simulink model "DS3or"  (R2023a)
settings: Solver=VariableStepAuto  StartTime=0.0  StopTime=tsim  RelTol=1e-3
undefined symbols (not defined in the file): comp_noise_rms, comp_offset, fclk, fin, fs, OSR, pf1, pf2, pf3, ps1, ps2, ps3, q1, q2, q3, VDD, Vin_amp, Vin_cm, Vin_DC, Vref, VSS, W
settings Model: Creator=amantilla  LastModifiedBy=alexm
settings SolverCC: AlgebraicLoopSolver=TrustRegion
settings DebuggingCC: UnconnectedInputMsg=warning  UnconnectedOutputMsg=warning  UnconnectedLineMsg=warning
settings ModelReferenceCC: EnableRefExpFcnMdlSchedulingChecks=on
settings RTWCC: DLArmComputeVersion=19.05

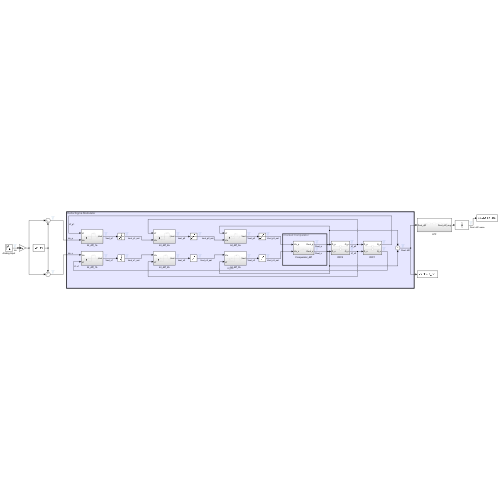
[thumbnail: Simulink's stored preview of the top-level diagram]
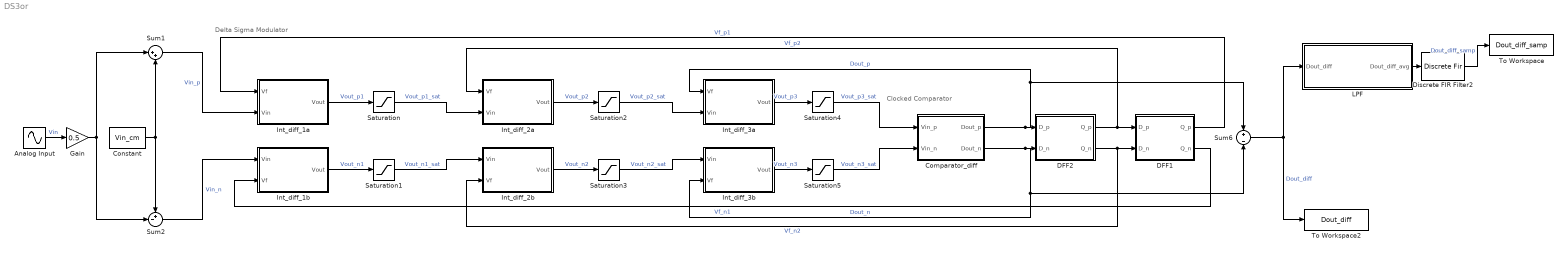
== system DS3or ==
  note: Delta Sigma Modulator
  note: Clocked Comparator
  Analog Input : Sin  Amplitude=Vin_amp  Bias=Vin_DC  Frequency=2*pi*fin  SampleTime=1/(fclk)
  Comparator_diff : Subsystem
  Constant : Constant  Value=Vin_cm
  DFF1 : Subsystem
  DFF2 : Subsystem
  Discrete FIR Filter2 : DiscreteFir  Coefficients=1  InitialStates=(VDD - VSS)/2  SampleTime=1/(fs)
  Gain : Gain  Gain=0.5
  Int_diff_1a : Subsystem
  Int_diff_1b : Subsystem
  Int_diff_2a : Subsystem
  Int_diff_2b : Subsystem
  Int_diff_3a : Subsystem
  Int_diff_3b : Subsystem
  LPF : Subsystem
  Saturation{,1..5} (6 alike) : Saturate  UpperLimit=0.9  LowerLimit=0
  Sum1 : Sum  Inputs=|++
  Sum2 : Sum  Inputs=+-|
  Sum6 : Sum  Inputs=+|-
  To Workspace : ToWorkspace  VariableName=Dout_diff_samp  SaveFormat=Timeseries  SampleTime=1/fs
  To Workspace2 : ToWorkspace  VariableName=Dout_diff  SaveFormat=Timeseries  SampleTime=1/fclk
  wires:
  Constant/1 -> Sum1/2, Sum2/1
  Sum6/1 -> To Workspace2/1, LPF/1(Dout_diff)  "Dout_diff"
  Gain/1 -> Sum2/2, Sum1/1
  Discrete FIR Filter2/1 -> To Workspace/1  "Dout_diff_samp"
  Sum2/1 -> Int_diff_1b/1(Vin)  "Vin_n"
  Int_diff_2b/1(Vout) -> Saturation3/1  "Vout_n2"
  Analog Input/1 -> Gain/1  "Vin"
  Sum1/1 -> Int_diff_1a/2(Vin)  "Vin_p"
  Int_diff_2a/1(Vout) -> Saturation2/1  "Vout_p2"
  Int_diff_1a/1(Vout) -> Saturation/1  "Vout_p1"
  Int_diff_1b/1(Vout) -> Saturation1/1  "Vout_n1"
  DFF1/1(Q_p) -> Int_diff_1a/1(Vf)  "Vf_p1"
  DFF1/2(Q_n) -> Int_diff_1b/2(Vf)  "Vf_n1"
  Comparator_diff/1(Dout_p) -> Sum6/1, Int_diff_3a/1(Vf), DFF2/1(D_p)  "Dout_p"
  Comparator_diff/2(Dout_n) -> Sum6/2, Int_diff_3b/2(Vf), DFF2/2(D_n)  "Dout_n"
  Saturation/1 -> Int_diff_2a/2(Vin)  "Vout_p1_sat"
  Saturation1/1 -> Int_diff_2b/1(Vin)  "Vout_n1_sat"
  Saturation2/1 -> Int_diff_3a/2(Vin)  "Vout_p2_sat"
  Saturation3/1 -> Int_diff_3b/1(Vin)  "Vout_n2_sat"
  DFF2/1(Q_p) -> DFF1/1(D_p), Int_diff_2a/1(Vf)  "Vf_p2"
  DFF2/2(Q_n) -> DFF1/2(D_n), Int_diff_2b/2(Vf)  "Vf_n2"
  Int_diff_3b/1(Vout) -> Saturation5/1  "Vout_n3"
  Int_diff_3a/1(Vout) -> Saturation4/1  "Vout_p3"
  Saturation4/1 -> Comparator_diff/1(Vin_p)  "Vout_p3_sat"
  Saturation5/1 -> Comparator_diff/2(Vin_n)  "Vout_n3_sat"
  LPF/1(Dout_diff_avg) -> Discrete FIR Filter2/1

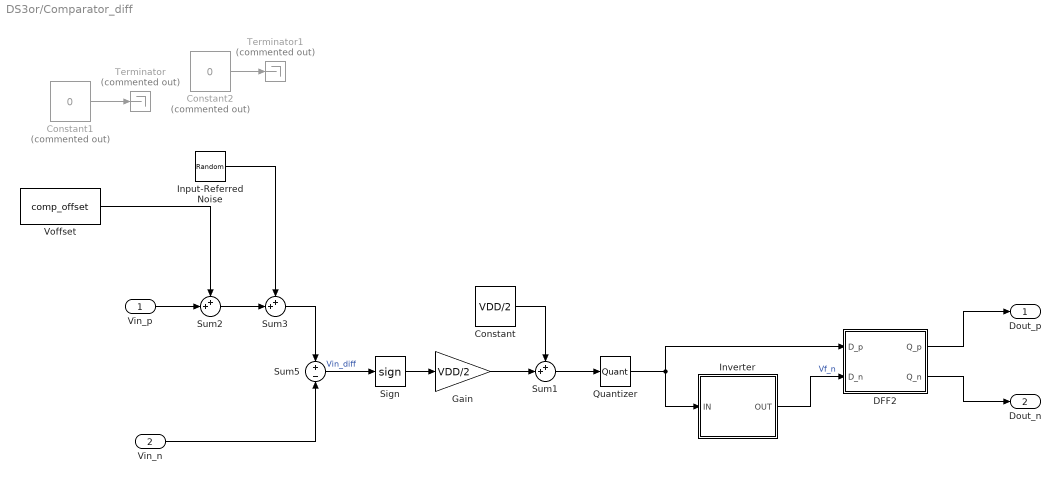
== system DS3or/Comparator_diff ==
  Vin_p : Inport
  Vin_n : Inport  Port=2
  Constant : Constant  Value=VDD/2  VectorParams1D=off  SampleTime=-1
  Constant1 : Constant  Commented=on  Value=0  VectorParams1D=off  SampleTime=-1
  Constant2 : Constant  Commented=on  Value=0  VectorParams1D=off  SampleTime=-1
  DFF2 : Subsystem
  Gain : Gain  Gain=VDD/2
  Input-Referred Noise : RandomNumber  Variance=comp_noise_rms  SampleTime=1/(4*fclk)
  Inverter : Subsystem
  Quantizer : Quantizer  QuantizationInterval=(VDD-VSS)
  Sign : Signum
  Sum1 : Sum  Inputs=++|
  Sum2 : Sum  Inputs=++|
  Sum3 : Sum  Inputs=++|
  Sum5 : Sum  Inputs=+|-
  Terminator : Terminator  Commented=on
  Terminator1 : Terminator  Commented=on
  Voffset : Constant  Value=comp_offset  VectorParams1D=off  SampleTime=-1
  Dout_p : Outport
  Dout_n : Outport  Port=2
  wires:
  Sum5/1 -> Sign/1  "Vin_diff"
  Vin_n/1 -> Sum5/2
  Sign/1 -> Gain/1
  Gain/1 -> Sum1/2
  Sum1/1 -> Quantizer/1
  Constant/1 -> Sum1/1
  Inverter/1(OUT) -> DFF2/2(D_n)  "Vf_n"
  Quantizer/1 -> Inverter/1(IN), DFF2/1(D_p)
  DFF2/1(Q_p) -> Dout_p/1
  DFF2/2(Q_n) -> Dout_n/1
  Vin_p/1 -> Sum2/2
  Sum2/1 -> Sum3/2
  Sum3/1 -> Sum5/1
  Constant1/1 -> Terminator/1
  Constant2/1 -> Terminator1/1
  Input-Referred Noise/1 -> Sum3/1
  Voffset/1 -> Sum2/1

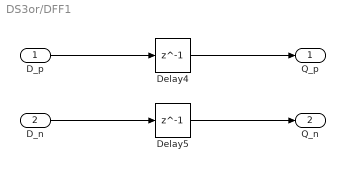
== system DS3or/DFF1 ==
  D_p : Inport
  D_n : Inport  Port=2
  Delay4 : Delay  DelayLength=1  InitialCondition=VSS  SampleTime=1/(fclk)
  Delay5 : Delay  DelayLength=1  InitialCondition=VDD  SampleTime=1/(fclk)
  Q_p : Outport
  Q_n : Outport  Port=2
  wires:
  Delay4/1 -> Q_p/1
  D_p/1 -> Delay4/1
  Delay5/1 -> Q_n/1
  D_n/1 -> Delay5/1

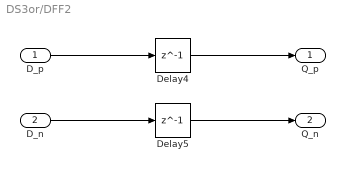
== system DS3or/DFF2 ==
  D_p : Inport
  D_n : Inport  Port=2
  Delay4 : Delay  DelayLength=1  InitialCondition=VSS  SampleTime=1/(fclk)
  Delay5 : Delay  DelayLength=1  InitialCondition=VDD  SampleTime=1/(fclk)
  Q_p : Outport
  Q_n : Outport  Port=2
  wires:
  Delay4/1 -> Q_p/1
  D_p/1 -> Delay4/1
  Delay5/1 -> Q_n/1
  D_n/1 -> Delay5/1

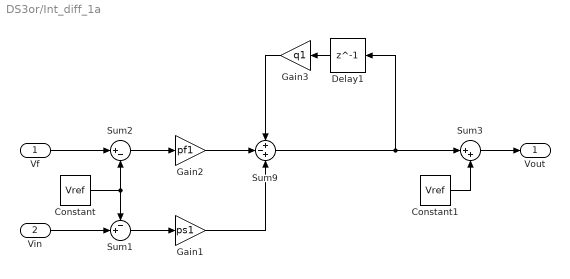
== system DS3or/Int_diff_1a ==
  Vf : Inport
  Vin : Inport  Port=2
  Constant : Constant  Value=Vref
  Constant1 : Constant  Value=Vref
  Delay1 : Delay  DelayLength=1  SampleTime=1/(fclk)
  Gain1 : Gain  Gain=ps1
  Gain2 : Gain  Gain=pf1
  Gain3 : Gain  Gain=q1
  Sum1 : Sum  Inputs=-+|
  Sum2 : Sum  Inputs=|+-
  Sum3 : Sum  Inputs=|++
  Sum9 : Sum  Inputs=+-+
  Vout : Outport
  wires:
  Vf/1 -> Sum2/1
  Vin/1 -> Sum1/2
  Constant/1 -> Sum2/2, Sum1/1
  Sum2/1 -> Gain2/1
  Sum1/1 -> Gain1/1
  Gain2/1 -> Sum9/2
  Gain1/1 -> Sum9/3
  Constant1/1 -> Sum3/2
  Sum3/1 -> Vout/1
  Sum9/1 -> Delay1/1, Sum3/1
  Delay1/1 -> Gain3/1
  Gain3/1 -> Sum9/1

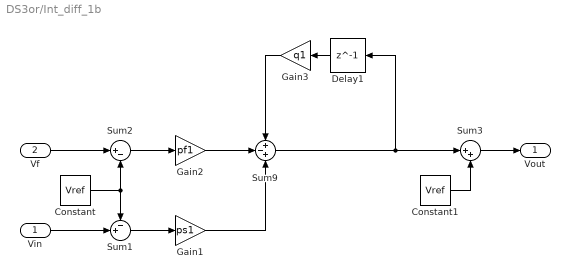
== system DS3or/Int_diff_1b ==
  Vin : Inport
  Vf : Inport  Port=2
  Constant : Constant  Value=Vref
  Constant1 : Constant  Value=Vref
  Delay1 : Delay  DelayLength=1  SampleTime=1/(fclk)
  Gain1 : Gain  Gain=ps1
  Gain2 : Gain  Gain=pf1
  Gain3 : Gain  Gain=q1
  Sum1 : Sum  Inputs=-+|
  Sum2 : Sum  Inputs=|+-
  Sum3 : Sum  Inputs=|++
  Sum9 : Sum  Inputs=+-+
  Vout : Outport
  wires:
  Vf/1 -> Sum2/1
  Vin/1 -> Sum1/2
  Constant/1 -> Sum2/2, Sum1/1
  Sum2/1 -> Gain2/1
  Sum1/1 -> Gain1/1
  Gain2/1 -> Sum9/2
  Gain1/1 -> Sum9/3
  Constant1/1 -> Sum3/2
  Sum3/1 -> Vout/1
  Sum9/1 -> Delay1/1, Sum3/1
  Delay1/1 -> Gain3/1
  Gain3/1 -> Sum9/1

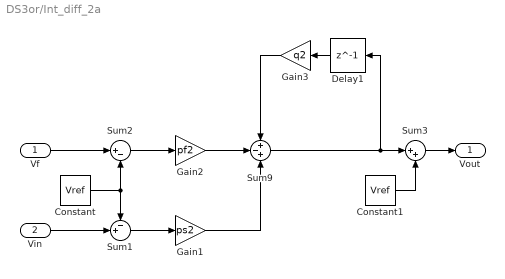
== system DS3or/Int_diff_2a ==
  Vf : Inport
  Vin : Inport  Port=2
  Constant : Constant  Value=Vref
  Constant1 : Constant  Value=Vref
  Delay1 : Delay  DelayLength=1  SampleTime=1/(fclk)
  Gain1 : Gain  Gain=ps2
  Gain2 : Gain  Gain=pf2
  Gain3 : Gain  Gain=q2
  Sum1 : Sum  Inputs=-+|
  Sum2 : Sum  Inputs=|+-
  Sum3 : Sum  Inputs=|++
  Sum9 : Sum  Inputs=+-+
  Vout : Outport
  wires:
  Vf/1 -> Sum2/1
  Vin/1 -> Sum1/2
  Constant/1 -> Sum2/2, Sum1/1
  Sum2/1 -> Gain2/1
  Sum1/1 -> Gain1/1
  Gain2/1 -> Sum9/2
  Gain1/1 -> Sum9/3
  Constant1/1 -> Sum3/2
  Sum3/1 -> Vout/1
  Sum9/1 -> Sum3/1, Delay1/1
  Delay1/1 -> Gain3/1
  Gain3/1 -> Sum9/1

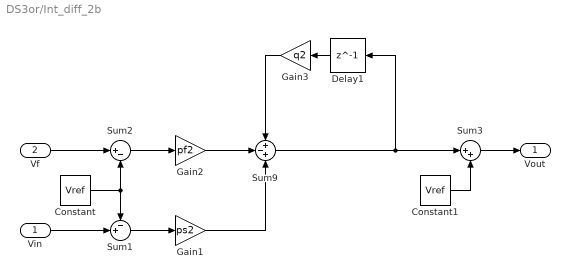
== system DS3or/Int_diff_2b ==
  Vin : Inport
  Vf : Inport  Port=2
  Constant : Constant  Value=Vref
  Constant1 : Constant  Value=Vref
  Delay1 : Delay  DelayLength=1  SampleTime=1/(fclk)
  Gain1 : Gain  Gain=ps2
  Gain2 : Gain  Gain=pf2
  Gain3 : Gain  Gain=q2
  Sum1 : Sum  Inputs=-+|
  Sum2 : Sum  Inputs=|+-
  Sum3 : Sum  Inputs=|++
  Sum9 : Sum  Inputs=+-+
  Vout : Outport
  wires:
  Vf/1 -> Sum2/1
  Vin/1 -> Sum1/2
  Constant/1 -> Sum2/2, Sum1/1
  Sum2/1 -> Gain2/1
  Sum1/1 -> Gain1/1
  Gain2/1 -> Sum9/2
  Gain1/1 -> Sum9/3
  Constant1/1 -> Sum3/2
  Sum3/1 -> Vout/1
  Sum9/1 -> Delay1/1, Sum3/1
  Delay1/1 -> Gain3/1
  Gain3/1 -> Sum9/1

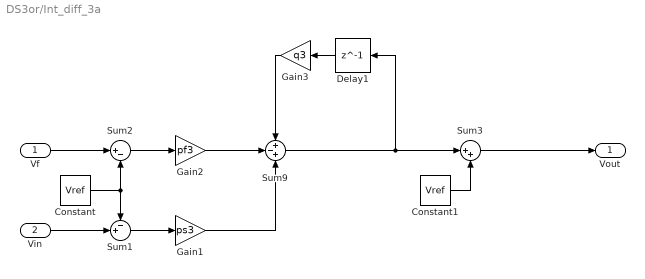
== system DS3or/Int_diff_3a ==
  Vf : Inport
  Vin : Inport  Port=2
  Constant : Constant  Value=Vref
  Constant1 : Constant  Value=Vref
  Delay1 : Delay  DelayLength=1  SampleTime=1/(fclk)
  Gain1 : Gain  Gain=ps3
  Gain2 : Gain  Gain=pf3
  Gain3 : Gain  Gain=q3
  Sum1 : Sum  Inputs=-+|
  Sum2 : Sum  Inputs=|+-
  Sum3 : Sum  Inputs=|++
  Sum9 : Sum  Inputs=+-+
  Vout : Outport
  wires:
  Vf/1 -> Sum2/1
  Vin/1 -> Sum1/2
  Constant/1 -> Sum2/2, Sum1/1
  Sum2/1 -> Gain2/1
  Sum1/1 -> Gain1/1
  Gain2/1 -> Sum9/2
  Gain1/1 -> Sum9/3
  Constant1/1 -> Sum3/2
  Sum3/1 -> Vout/1
  Sum9/1 -> Delay1/1, Sum3/1
  Delay1/1 -> Gain3/1
  Gain3/1 -> Sum9/1

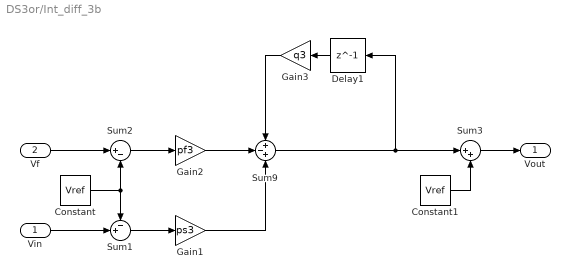
== system DS3or/Int_diff_3b ==
  Vin : Inport
  Vf : Inport  Port=2
  Constant : Constant  Value=Vref
  Constant1 : Constant  Value=Vref
  Delay1 : Delay  DelayLength=1  SampleTime=1/(fclk)
  Gain1 : Gain  Gain=ps3
  Gain2 : Gain  Gain=pf3
  Gain3 : Gain  Gain=q3
  Sum1 : Sum  Inputs=-+|
  Sum2 : Sum  Inputs=|+-
  Sum3 : Sum  Inputs=|++
  Sum9 : Sum  Inputs=+-+
  Vout : Outport
  wires:
  Vf/1 -> Sum2/1
  Vin/1 -> Sum1/2
  Constant/1 -> Sum2/2, Sum1/1
  Sum2/1 -> Gain2/1
  Sum1/1 -> Gain1/1
  Gain2/1 -> Sum9/2
  Gain1/1 -> Sum9/3
  Constant1/1 -> Sum3/2
  Sum3/1 -> Vout/1
  Sum9/1 -> Delay1/1, Sum3/1
  Delay1/1 -> Gain3/1
  Gain3/1 -> Sum9/1

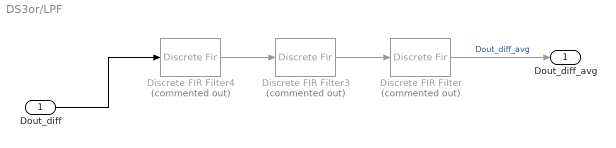
== system DS3or/LPF ==
  Dout_diff : Inport
  Discrete FIR Filter : DiscreteFir  Commented=on  Coefficients=W  InitialStates=(VDD - VSS)/2  SampleTime=1/(fs*OSR)
  Discrete FIR Filter3 : DiscreteFir  Commented=on  Coefficients=W  InitialStates=(VDD - VSS)/2  SampleTime=1/(fs*OSR)
  Discrete FIR Filter4 : DiscreteFir  Commented=on  Coefficients=W  InitialStates=(VDD - VSS)/2  SampleTime=1/(fs*OSR)
  Dout_diff_avg : Outport
  wires:
  Discrete FIR Filter4/1 -> Discrete FIR Filter3/1
  Discrete FIR Filter3/1 -> Discrete FIR Filter/1
  Discrete FIR Filter/1 -> Dout_diff_avg/1  "Dout_diff_avg"
  Dout_diff/1 -> Discrete FIR Filter4/1

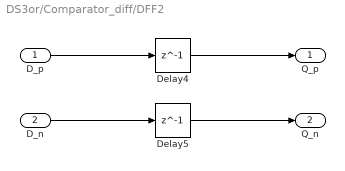
== system DS3or/Comparator_diff/DFF2 ==
  D_p : Inport
  D_n : Inport  Port=2
  Delay4 : Delay  DelayLength=1  InitialCondition=VSS  SampleTime=1/(fclk)
  Delay5 : Delay  DelayLength=1  InitialCondition=VDD  SampleTime=1/(fclk)
  Q_p : Outport
  Q_n : Outport  Port=2
  wires:
  Delay4/1 -> Q_p/1
  D_p/1 -> Delay4/1
  Delay5/1 -> Q_n/1
  D_n/1 -> Delay5/1

== system DS3or/Comparator_diff/Inverter ==
  IN : Inport
  Constant : Constant  Value=VDD
  Sum1 : Sum  Inputs=+-|
  OUT : Outport
  wires:
  Sum1/1 -> OUT/1  "Vf_n"
  IN/1 -> Sum1/2
  Constant/1 -> Sum1/1
